simulink model "FederatedSystem"  (R2023b)
settings: Solver=FixedStepAuto  StartTime=0.0  StopTime=Inf  RelTol=1e-3
settings Model: Creator=bubuk  LastModifiedBy=bubuk
settings ConfigComp: DVMode=PropertyProving  DVTestSuiteOptimization=Auto  DVDetectOutOfBounds=on  DVModelReferenceHarness=on  DVHarnessSource=Signal Editor  DVRebuildModelRepresentation=IfChangeIsDetected

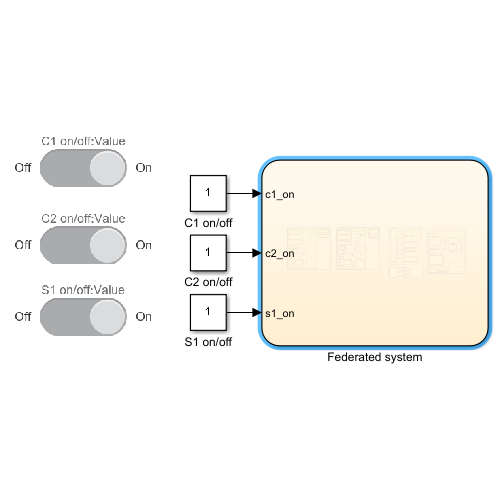
[thumbnail: Simulink's stored preview of the top-level diagram]
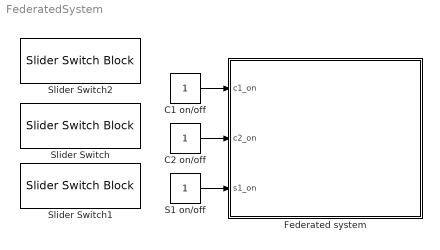
== system FederatedSystem ==
  C1 on/off : Constant
  C2 on/off : Constant
  Federated system : Stateflow chart  TreatAsAtomicUnit=on
  S1 on/off : Constant
  Slider Switch : SliderSwitchBlock
      settings: Values={{'Off', 'On'}, [0 1]}
  Slider Switch1 : SliderSwitchBlock
      settings: Values={{'Off', 'On'}, [0 1]}
  Slider Switch2 : SliderSwitchBlock
      settings: Values={{'Off', 'On'}, [0 1]}
  wires:
  C2 on/off/1 -> Federated system/2(c2_on)
  S1 on/off/1 -> Federated system/3(s1_on)
  C1 on/off/1 -> Federated system/1(c1_on)

== stateflow chart FederatedSystem/Federated system ==
  state Database [parallel]
    settings: executionOrder=3
    state DATABASE_INTERFACE
    state CONFIGURATION
      entry:
      C_configuration.data = C_getConfiguration.data
      exit:
      send(C_configuration)
      switch C_getConfiguration.data
      case "client1"
      send(configuration,Client_1_box.Client_1.INIT.WAIT_FOR_CONFIGURATION)
      case "client2"
      send(configuration,Client_2_box.Client_2.INIT.WAIT_FOR_CONFIGURATION)
      end
    state SERVER_SELECTION
      entry:
      switch C_serverSelection.data
      case "server1"
      if c1_on ==1 && c2_on ==1
      s1_clients =2;
      else s1_clients=1
      end
      end
    state JOB
      entry:
      if c1_state == "wait_for_job"
      send(S1_sendJob,Client_1_box.Client_1.READY.WAIT_FOR_JOB)
      end
      if c2_state == "wait_for_job"
      send(S1_sendJob,Client_2_box.Client_2.READY.WAIT_FOR_JOB)
      end
    state LOCAL_MODEL
      entry:
      send(C_localWeights,Server__box.Server_1)
    state GLOBAL_MODEL
      entry:
      if c1_state == "model_trained"
      send(S1_globalWeights,Client_1_box.Client_1.WAIT_FOR_DATA)
      end
      if c2_state == "model_trained"
      send(S1_globalWeights,Client_2_box.Client_2.WAIT_FOR_DATA)
      end
    state GLOBAL_MODEL1
      entry:
      send(S_globalModel,Client_1_box.Client_1.RESTORE)
      send(S_globalModel,Client_2_box.Client_2.RESTORE)
    DATABASE_INTERFACE -> Database.CONFIGURATION [order 1] : C_getConfiguration
    Database.CONFIGURATION -> DATABASE_INTERFACE
    (default) -> DATABASE_INTERFACE
    DATABASE_INTERFACE -> SERVER_SELECTION [order 2] : C_serverSelection
    SERVER_SELECTION -> DATABASE_INTERFACE
    DATABASE_INTERFACE -> JOB [order 3] : S1_sendJob
    JOB -> DATABASE_INTERFACE
    DATABASE_INTERFACE -> LOCAL_MODEL [order 4] : C_localWeights
    LOCAL_MODEL -> DATABASE_INTERFACE
    DATABASE_INTERFACE -> GLOBAL_MODEL [order 5] : S1_globalWeights
    GLOBAL_MODEL -> DATABASE_INTERFACE
    DATABASE_INTERFACE -> GLOBAL_MODEL1 [order 6] : C_getGlobalModel
    GLOBAL_MODEL1 -> DATABASE_INTERFACE
  state Client_2_box [group]
    state Client_2 [parallel]
      settings: executionOrder=1
      state INIT
        state READY
          entry:
          c2_state = "online"
          exit:
          C_getConfiguration.data = "client2"
          send(C_getConfiguration)
          send(C2_getConfiguration,Database)
        state WAIT_FOR_CONFIGURATION
          entry,during:
          c2_state = "wait_for_configuration"
          if receive(C_configuration) && C_configuration.data == "client2"
          c2_set_configuration = true
          c2_model_version = s1_model_version
          c2_model_ready = true
          end
        Client_2_box.Client_2.INIT.READY -> Client_2_box.Client_2.INIT.WAIT_FOR_CONFIGURATION [order 2] : [c2_on==1]
        Client_2_box.Client_2.INIT.WAIT_FOR_CONFIGURATION -> Client_2_box.Client_2.INIT.READY [order 2] : after(60,sec)
      state OFF
        entry:
        if c2_set_configuration == true
        s1_clients = s1_clients - 1;
        c2_set_configuration = false;
        end
      state CONFIGURATION
        entry:
        c2_state = "configuration"
        exit:
        C_serverSelection.data = "server1"
        send(C_serverSelection)
        send(C2_serverSelection,Database)
      state READY
        state READY_TO_JOB
          entry:
          c2_state = "ready"
          send(C2_readyToJob,Database)
        state WAIT_FOR_JOB
          entry,during:
          c2_state = "wait_for_job"
          if s1_state== "send_job"
          c2_job = true;
          c2_rounds = 0;
          end
        Client_2_box.Client_2.READY.READY_TO_JOB -> Client_2_box.Client_2.READY.WAIT_FOR_JOB [order 2] : [c2_on == 1]
      state RESTORE
        entry:
        c2_state = "restore"
        c2_model_ready = false;
        send (C_getGlobalModel,Database)
        during:
        if s1_model_version > c2_model_version
        c2_model_ready = true;
        c2_model_version = s1_model_version;
        end
      state GATHER_DATA
        entry:
        c2_state = "gather_data"
      state WAIT_FOR_DATA
        entry,during:
        c2_state = "model_trained"
        if c2_rounds == 3
        c2_job = false
        end
        if s1_state == "global_round_trained"
        c2_model_ready = true;
        end
      state TRAINING_MODEL
        state MODEL_TRAINED
          entry:
          c2_state = "model_trained"
          c2_rounds = c2_rounds + 1;
          c2_model_ready = false;
          send(C_localWeights,Database)
        state TRAINING
          entry:
          c2_state = "training"
        Client_2_box.Client_2.TRAINING_MODEL.TRAINING -> Client_2_box.Client_2.TRAINING_MODEL.MODEL_TRAINED : after(10,sec)
      (default) -> Client_2_box.Client_2.INIT.READY
      Client_2_box.Client_2.OFF -> Client_2_box.Client_2.INIT.READY : [c2_on==1]
      Client_2_box.Client_2.INIT.READY -> Client_2_box.Client_2.OFF [order 1] : [c2_on == 0]
      Client_2_box.Client_2.INIT.WAIT_FOR_CONFIGURATION -> Client_2_box.Client_2.OFF [order 1] : [c2_on == 0]
      Client_2_box.Client_2.CONFIGURATION -> Client_2_box.Client_2.OFF [order 1] : [c2_on == 0]
      (junction 612) -> Client_2_box.Client_2.OFF
      Client_2_box.Client_2.INIT -> Client_2_box.Client_2.CONFIGURATION : [c2_set_configuration == true]
      Client_2_box.Client_2.CONFIGURATION -> Client_2_box.Client_2.READY.READY_TO_JOB [order 2] : [c1_on == 1]
      Client_2_box.Client_2.RESTORE -> Client_2_box.Client_2.READY.READY_TO_JOB [order 2] : [c2_model_ready == true]
      Client_2_box.Client_2.READY.READY_TO_JOB -> (junction 612) [order 1] : [c2_on == 0]
      Client_2_box.Client_2.READY.WAIT_FOR_JOB -> (junction 612) [order 1] : [c2_on == 0]
      Client_2_box.Client_2.RESTORE -> (junction 612) [order 1] : [c2_on == 0]
      Client_2_box.Client_2.WAIT_FOR_DATA -> Client_2_box.Client_2.RESTORE [order 3] : [c2_job== false]
      Client_2_box.Client_2.READY.WAIT_FOR_JOB -> Client_2_box.Client_2.GATHER_DATA [order 2] : [c2_job == true]
      Client_2_box.Client_2.WAIT_FOR_DATA -> (junction 612) [order 1] : [c2_on == 0]
      Client_2_box.Client_2.TRAINING_MODEL.MODEL_TRAINED -> (junction 612) [order 1] : [c2_on == 0]
      Client_2_box.Client_2.GATHER_DATA -> Client_2_box.Client_2.TRAINING_MODEL.TRAINING : after(10,sec)
      Client_2_box.Client_2.TRAINING_MODEL.MODEL_TRAINED -> Client_2_box.Client_2.WAIT_FOR_DATA [order 2] : [c2_on == 1]
      Client_2_box.Client_2.WAIT_FOR_DATA -> Client_2_box.Client_2.TRAINING_MODEL.TRAINING [order 2] : [c2_model_ready == true]
    state Client_2_keepalive [parallel]
      settings: executionOrder=2
      state SENDING
        entry:
        if c1_on == true
        send(C2_keepAlive, Database_keepalive)
        end
      state WAITING
      (default) -> Client_2_box.Client_2_keepalive.SENDING
      Client_2_box.Client_2_keepalive.SENDING -> Client_2_box.Client_2_keepalive.WAITING
      Client_2_box.Client_2_keepalive.WAITING -> Client_2_box.Client_2_keepalive.SENDING : after(20,sec)
  state Client_1_box [group]
    state Client_1 [parallel]
      settings: executionOrder=1
      state INIT
        state READY
          entry:
          c1_state = "online"
          exit:
          C_getConfiguration.data = "client1"
          send(C_getConfiguration)
          send(C1_getConfiguration,Database)
        state WAIT_FOR_CONFIGURATION
          entry,during:
          c1_state = "wait_for_configuration"
          if receive(C_configuration) && C_configuration.data == "client1"
          c1_set_configuration = true
          c1_model_version = s1_model_version
          c1_model_ready = true
          end
        Client_1_box.Client_1.INIT.READY -> Client_1_box.Client_1.INIT.WAIT_FOR_CONFIGURATION [order 2] : [c1_on==1]
        Client_1_box.Client_1.INIT.WAIT_FOR_CONFIGURATION -> Client_1_box.Client_1.INIT.READY [order 2] : after(60,sec)
      state OFF
        entry:
        if c1_set_configuration == true
        s1_clients = s1_clients - 1;
        c1_set_configuration = false;
        end
      state CONFIGURATION
        entry:
        c1_state = "configuration"
        exit:
        C_serverSelection.data = "server1"
        send(C_serverSelection)
        send(C1_serverSelection,Database)
      state READY
        state READY_TO_JOB
          entry:
          c1_state = "ready"
          send(C1_readyToJob,Database)
        state WAIT_FOR_JOB
          entry,during:
          c1_state = "wait_for_job"
          if s1_state== "send_job"
          c1_job = true;
          c1_rounds = 0;
          end
        Client_1_box.Client_1.READY.READY_TO_JOB -> Client_1_box.Client_1.READY.WAIT_FOR_JOB [order 2] : [c1_on == 1]
      state RESTORE
        entry:
        c1_state = "restore"
        c1_model_ready = false;
        send (C_getGlobalModel,Database)
        during:
        if s1_model_version > c1_model_version
        c1_model_ready = true;
        c1_model_version = s1_model_version;
        end
      state GATHER_DATA
        entry:
        c1_state = "gather_data"
      state WAIT_FOR_DATA
        entry,during:
        c1_state = "model_trained"
        if c1_rounds == 3
        c1_job = false
        end
        if s1_state == "global_round_trained"
        c1_model_ready = true;
        end
      state TRAINING_MODEL
        state MODEL_TRAINED
          entry:
          c1_state = "model_trained"
          c1_rounds = c1_rounds + 1;
          c1_model_ready = false;
          send(C_localWeights,Database)
        state TRAINING
          entry:
          c1_state = "training"
        Client_1_box.Client_1.TRAINING_MODEL.TRAINING -> Client_1_box.Client_1.TRAINING_MODEL.MODEL_TRAINED : after(10,sec)
      Client_1_box.Client_1.OFF -> Client_1_box.Client_1.INIT.READY : [c1_on==1]
      Client_1_box.Client_1.INIT.READY -> Client_1_box.Client_1.OFF [order 1] : [c1_on == 0]
      Client_1_box.Client_1.INIT.WAIT_FOR_CONFIGURATION -> Client_1_box.Client_1.OFF [order 1] : [c1_on == 0]
      Client_1_box.Client_1.CONFIGURATION -> Client_1_box.Client_1.OFF [order 1] : [c1_on == 0]
      (junction 566) -> Client_1_box.Client_1.OFF
      Client_1_box.Client_1.INIT -> Client_1_box.Client_1.CONFIGURATION : [c1_set_configuration == true]
      Client_1_box.Client_1.CONFIGURATION -> Client_1_box.Client_1.READY.READY_TO_JOB [order 2] : [c1_on == 1]
      Client_1_box.Client_1.RESTORE -> Client_1_box.Client_1.READY.READY_TO_JOB [order 2] : [c1_model_ready == true]
      Client_1_box.Client_1.READY.READY_TO_JOB -> (junction 566) [order 1] : [c1_on == 0]
      Client_1_box.Client_1.READY.WAIT_FOR_JOB -> (junction 566) [order 1] : [c1_on == 0]
      Client_1_box.Client_1.RESTORE -> (junction 566) [order 1] : [c1_on == 0]
      Client_1_box.Client_1.WAIT_FOR_DATA -> Client_1_box.Client_1.RESTORE [order 3] : [c1_job== false]
      Client_1_box.Client_1.READY.WAIT_FOR_JOB -> Client_1_box.Client_1.GATHER_DATA [order 2] : [c1_job == true]
      Client_1_box.Client_1.WAIT_FOR_DATA -> (junction 566) [order 1] : [c1_on == 0]
      Client_1_box.Client_1.TRAINING_MODEL.MODEL_TRAINED -> (junction 566) [order 1] : [c1_on == 0]
      Client_1_box.Client_1.GATHER_DATA -> Client_1_box.Client_1.TRAINING_MODEL.TRAINING : after(10,sec)
      Client_1_box.Client_1.TRAINING_MODEL.MODEL_TRAINED -> Client_1_box.Client_1.WAIT_FOR_DATA [order 2] : [c1_on == 1]
      Client_1_box.Client_1.WAIT_FOR_DATA -> Client_1_box.Client_1.TRAINING_MODEL.TRAINING [order 2] : [c1_model_ready == true]
    state Client_1_keepalive [parallel]
      settings: executionOrder=2
      state SENDING
        entry:
        if c1_on == true
        send(C1_keepAlive, Database_keepalive)
        end
      state WAITING
      (default) -> Client_1_box.Client_1_keepalive.SENDING
      Client_1_box.Client_1_keepalive.SENDING -> Client_1_box.Client_1_keepalive.WAITING
      Client_1_box.Client_1_keepalive.WAITING -> Client_1_box.Client_1_keepalive.SENDING : after(20,sec)
  state Server__box [group]
    state Server_1 [parallel]
      settings: executionOrder=1
      state MODEL
        entry:
        s1_state = "online";
        exit:
        s1_model_version = s1_model_version+1;
      state SERVER_INTERFACE
        entry,during:
        s1_state = "waiting_for_clients";
        s1_clients_ready=0;
        if (c1_state== "wait_for_job")
        s1_clients_ready = s1_clients_ready + 1;
        end
        if (c2_state == "wait_for_job")
        s1_clients_ready = s1_clients_ready + 1;
        end
        if (s1_clients_ready==s1_clients && s1_clients_ready>0)
        s1_ready_to_job = true;
        end
      state TRAINING
        state GLOBAL_MODEL_TRAINED
          entry:
          s1_state = "global_model_trained"
          s1_model_version = s1_model_version + 1;
          send(S_globalModel,Database)
          exit:
          s1_client_weights=0;
          s1_ready_to_job = false;
        state TRAINING_GLOBAL_MODEL
          entry:
          s1_state = "global_round_trained"
          s1_ready_to_train = false;
          exit:
          send(S1_globalWeights,Database)
        TRAINING_GLOBAL_MODEL -> GLOBAL_MODEL_TRAINED [order 1] : [s1_rounds==3]
      state INITIALIZATION
        state SEND_JOB
          entry:
          s1_state = "send_job"
          s1_rounds=0;
          send(S1_sendJob,Database)
        state RECIEVE_JOBS
          entry,during:
          s1_client_weights=0;
          if c1_state== "model_trained"
          s1_client_weights = s1_client_weights + 1;
          end
          if c2_state == "model_trained"
          s1_client_weights = s1_client_weights + 1;
          end
          if s1_client_weights == s1_clients
          s1_ready_to_train = true;
          s1_rounds = s1_rounds + 1;
          send(S1_ready_to_train,Database);
          end
        SEND_JOB -> RECIEVE_JOBS : C_localWeights
      (default) -> MODEL
      MODEL -> SERVER_INTERFACE
      GLOBAL_MODEL_TRAINED -> SERVER_INTERFACE
      RECIEVE_JOBS -> GLOBAL_MODEL_TRAINED [order 2] : [c1_state == "restore"]
      SERVER_INTERFACE -> SEND_JOB : [s1_ready_to_job == true]
      TRAINING_GLOBAL_MODEL -> RECIEVE_JOBS [order 2] : after(10,sec)
      RECIEVE_JOBS -> TRAINING_GLOBAL_MODEL [order 1] : [s1_ready_to_train == true]
    state Server_1_keepalive [parallel]
      settings: executionOrder=2
      state SENDING
        entry:
        if s1_on == 1
        send(S1_keepAlive, Database_keepalive)
        end
      state WAITING
      Server__box.Server_1_keepalive.SENDING -> Server__box.Server_1_keepalive.WAITING
      (default) -> Server__box.Server_1_keepalive.SENDING
      Server__box.Server_1_keepalive.WAITING -> Server__box.Server_1_keepalive.SENDING : after(10,sec)
  state Database_keepalive [parallel]
    settings: executionOrder=2
    state SERVER1_STATE
      exit:
      s1_keep_alive = 30;
    state RECIEVE
      entry:
      if c1_keep_alive > 0
      c1_keep_alive = c1_keep_alive-1;
      else
      c1_state ="offline";
      end
      if c2_keep_alive > 0
      c2_keep_alive = c2_keep_alive-1;
      else
      c2_state ="offline";
      end
      if s1_keep_alive > 0
      s1_keep_alive = s1_keep_alive-1;
      else
      s1_state ="offline";
      end
    state CLIENT1_STATE
      exit:
      c1_keep_alive = 30;
    state CLIENT2_STATE
      exit:
      c2_keep_alive = 30;
    RECIEVE -> RECIEVE [order 4] : after(1,sec)
    RECIEVE -> SERVER1_STATE [order 1] : S1_keepAlive
    SERVER1_STATE -> RECIEVE
    (default) -> RECIEVE
    RECIEVE -> CLIENT1_STATE [order 2] : C1_keepAlive
    CLIENT1_STATE -> RECIEVE
    RECIEVE -> CLIENT2_STATE [order 3] : C2_keepAlive
    CLIENT2_STATE -> RECIEVE
  (default) -> Client_1_box.Client_1.INIT.READY
  data: c1_set_configuration local boolean =false; c1_model_ready local =false; c1_model_version local int64 =0; c1_state local string; c1_keep_alive local uint8 =0; s1_model_version local int64 =0; C_getConfiguration local string; C_configuration local string; c2_model_version local int64 =0; c2_model_ready local boolean =false; c2_set_configuration local boolean =false; s1_clients_ready local double =0; c2_state local string; c2_keep_alive local int8 =0; s1_keep_alive local int8 =0; s1_state local string; c1_job local boolean =false; c1_rounds local int8 =0; s1_clients local int8 =0; s1_ready_to_job local boolean =false; s1_client_weights local int8 =0; s1_ready_to_train local boolean =0; s1_rounds local int8 =0; c1_on input double =false; c2_on input double; s1_on input double; c2_rounds local int8 =0; c2_job local boolean =false; C_serverSelection local string
  events: C2_keepAlive local FUNCTION_CALL_EVENT; C1_keepAlive local FUNCTION_CALL_EVENT; S1_keepAlive local FUNCTION_CALL_EVENT; configuration local FUNCTION_CALL_EVENT; S1_sendJob local FUNCTION_CALL_EVENT; S_globalModel local FUNCTION_CALL_EVENT; S1_ready_to_train local FUNCTION_CALL_EVENT; C1_getConfiguration local FUNCTION_CALL_EVENT; C1_serverSelection local FUNCTION_CALL_EVENT; C1_readyToJob local FUNCTION_CALL_EVENT; C2_serverSelection local FUNCTION_CALL_EVENT; C2_readyToJob local FUNCTION_CALL_EVENT; C2_getConfiguration local FUNCTION_CALL_EVENT; S1_globalWeights local FUNCTION_CALL_EVENT; C_localWeights local FUNCTION_CALL_EVENT; C_getGlobalModel local FUNCTION_CALL_EVENT
